simulink model "plant"  (R2023a)
settings: Solver=ode4  StartTime=0.0  StopTime=t_duration  FixedStep=dt  RelTol=1e-3
undefined symbols (not defined in the file): plant
settings Model: Creator=ndelurgio  LastModifiedBy=ndelurgio

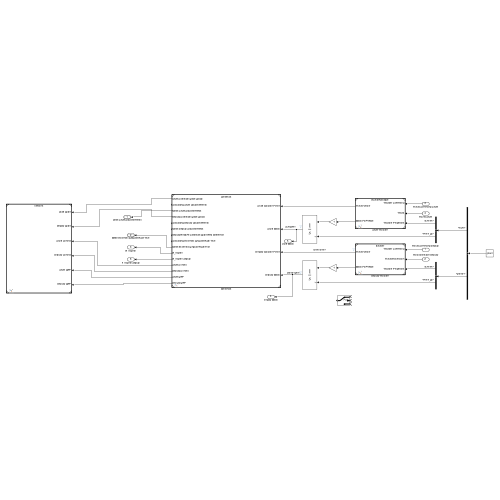
[thumbnail: Simulink's stored preview of the top-level diagram]
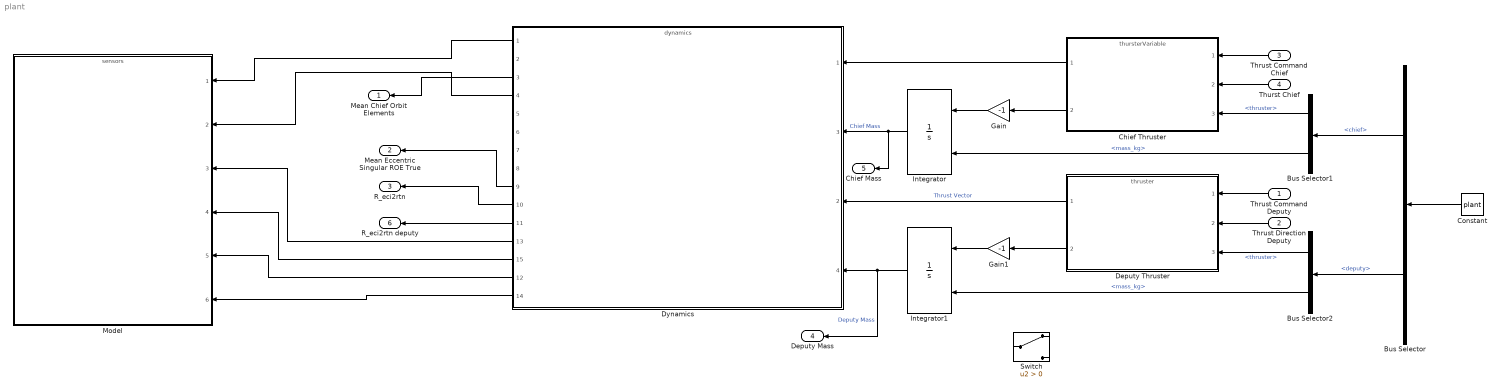
== system plant ==
  Thrust Command Deputy : Inport
  Thrust Direction Deputy : Inport  Port=2
  Thrust Command Chief : Inport  Port=3
  Thurst Chief : Inport  Port=4
  Bus Selector : BusSelector  OutputSignals=chief,deputy
  Bus Selector1 : BusSelector  OutputSignals=properties.actuators.thruster,initialConditions.mass_kg
  Bus Selector2 : BusSelector  OutputSignals=properties.actuators.thruster,initialConditions.mass_kg
  Chief Thruster : ModelReference  ModelNameDialog=thursterVariable.slx  SimulationMode=Normal  ModelReferenceVersion=1.4
  Constant : Constant  Value=plant  OutDataTypeStr=Bus: plantBus
  Deputy Thruster : ModelReference  ModelNameDialog=thruster.slx  SimulationMode=Normal  ModelReferenceVersion=1.13
  Dynamics : ModelReference  ModelNameDialog=dynamics.slx  SimulationMode=Normal  ModelReferenceVersion=1.204
      settings: PortSchema="{\"entries\":[{\"content\":{\"sides\":[{\"content\":{\"connectorIds\":[\"In1\",\"In3\",\"In2\",\"In4\"]},\"type\":\"ConnectorPlacement.EquallySpacedRectSide\",\"uuid\":\"856215f0-1594-44c2-a7bc-78e77c44fffd\"},{\"content\":{\"connectorIds\":[\"Out1\",\"Out2\",\"Out3\",\"Out4\",\"Out5\",\"Out6\",\"Out7\",\"Out8\",\"Out9\",\"Out10\",\"Out11\",\"Out13\",\"Out15\",\"Out12\",\"Out14\"],\"side\":\"RIGHT\"},\"type\":\"ConnectorPlacement.EquallySpacedRectSide\",\"uuid\":\"d770fffb-9e3a-4edd-82bb-f9465d0721e8\"},{\"content\":{\"side\":\"TOP\"},\"type\":\"ConnectorPlacement.EquallySpacedRectSide\",\"uuid\":\"c36e6b8f-cb45-4bbc-aa9c-a9462baed456\"}]},\"type\":\"ConnectorPlacement.EquallySpacedConnector\",\"uuid\":\"3ec004a9-95df-4d7e-ac6d-e27b9e7004e9\"}],\"packageUris\":[\"http://schema.mathworks.com/mf0/Connector/R2020b\"],\"version\":\"1.0\"}"
  Gain : Gain  Gain=-1
  Gain1 : Gain  Gain=-1
  Integrator : Integrator  InitialConditionSource=external
  Integrator1 : Integrator  InitialConditionSource=external
  Model : ModelReference  ModelNameDialog=sensors  SimulationMode=Normal  ModelReferenceVersion=1.4
  Switch : Switch  Criteria=u2 > Threshold  SaturateOnIntegerOverflow=off  InputSameDT=off
  Mean Chief Orbit Elements : Outport  OutDataTypeStr=Bus: meanOrbitElements
  Mean Eccentric Singular ROE True : Outport  Port=2  OutDataTypeStr=Bus: eccentricSingularROE
  R_eci2rtn : Outport  Port=3
  Deputy Mass : Outport  Port=4
  Chief Mass : Outport  Port=5
  R_eci2rtn deputy : Outport  Port=6
  wires:
  Chief Thruster/1 -> Dynamics/1
  Deputy Thruster/1 -> Dynamics/2  "Thrust Vector"
  Thrust Command Chief/1 -> Chief Thruster/1
  Thurst Chief/1 -> Chief Thruster/2
  Constant/1 -> Bus Selector/1
  Bus Selector/1 -> Bus Selector1/1  "<chief>"
  Bus Selector/2 -> Bus Selector2/1  "<deputy>"
  Chief Thruster/2 -> Gain/1
  Bus Selector1/1 -> Chief Thruster/3  "<thruster>"
  Bus Selector1/2 -> Integrator/2  "<mass_kg>"
  Bus Selector2/1 -> Deputy Thruster/3  "<thruster>"
  Bus Selector2/2 -> Integrator1/2  "<mass_kg>"
  Deputy Thruster/2 -> Gain1/1
  Integrator/1 -> Chief Mass/1, Dynamics/3  "Chief Mass"
  Integrator1/1 -> Deputy Mass/1, Dynamics/4  "Deputy Mass"
  Thrust Command Deputy/1 -> Deputy Thruster/1
  Thrust Direction Deputy/1 -> Deputy Thruster/2
  Dynamics/9 -> Mean Eccentric Singular ROE True/1
  Dynamics/10 -> R_eci2rtn/1
  Gain/1 -> Integrator/1
  Gain1/1 -> Integrator1/1
  Dynamics/3 -> Mean Chief Orbit Elements/1
  Dynamics/11 -> R_eci2rtn deputy/1
  Dynamics/1 -> Model/1
  Dynamics/4 -> Model/2
  Dynamics/13 -> Model/3
  Dynamics/12 -> Model/5
  Dynamics/15 -> Model/4
  Dynamics/14 -> Model/6
